simulink model "examplePVGenerator"  (R2013b)
settings: Solver=ode45  StartTime=0.0  StopTime=365*24*3600  RelTol=1e-3
libraries: carnot x3
settings Model: Creator=drhf  LastModifiedBy=drhf
settings OptimizationCC: ExpressionDepthLimit=2147483647
settings DebuggingCC: StateNameClashWarn=warning
settings GRTTargetCC: CombineOutputUpdateFcns=off  GRTInterface=on

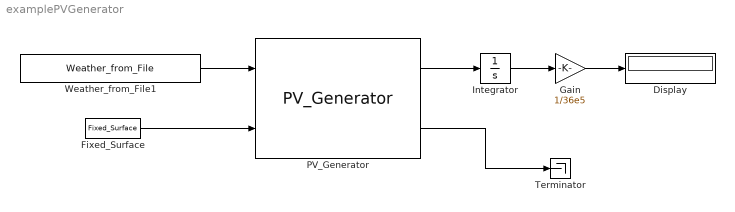
== system examplePVGenerator ==
  Display : Display
  Fixed_Surface : carnot/Weather/Fixed_Surface  colangle=30  colazi=0  colrot=0
  Gain : Gain  Gain=1/36e5
  Integrator : Integrator
  PV_Generator : carnot/Source/Electric_Generator/PV_Generator  Wp=1000  delta_Wp_K=0.0047  fgen=0.91 % 0.06 power missmatch, 0.01 diodes, 0.02 data sheet tolerance
  Terminator : Terminator
  Weather_from_File1 : carnot/Weather/Weather_from_File  file=DE_TRY2010_13_averageYear  ext=.mat
  wires:
  Weather_from_File1/1 -> PV_Generator/1
  Fixed_Surface/1 -> PV_Generator/2
  Integrator/1 -> Gain/1
  PV_Generator/1 -> Integrator/1
  Gain/1 -> Display/1
  PV_Generator/2 -> Terminator/1
